simulink model "pfb_legacy"  (Simulink 6.2)
settings: Solver=ode45  StartTime=0.0  StopTime=40000  RelTol=1e-3
undefined symbols (not defined in the file): BEE2_usr
libraries: xbsIndex_r3 x189, xps_library x42, adcscope_lib x6, pfb_library x3, fft_library x3, correlator_library x3
(part 2 of 2)

== system pfb_legacy/data_mux_in/tvg ==
  note: BRAM READ/WRITE MUX
      | lspitler - 13 Jan 09
      | Simplified TVG
      | tvg_ctrl sets 'length', 'skip', 'stall'
  Constant : xbsIndex_r3/Constant  const=0  equ=P=C  arith_type=Unsigned  n_bits=32  bin_pt=0  opselect=C  inp2=PCIN>>17  opr=+  inp1=P  carry=CIN  iostate=0  explicit_period=on  period=1  dbl_ovrd=off
  Constant1 : xbsIndex_r3/Constant  const=0  equ=P=C  arith_type=Unsigned  n_bits=32  bin_pt=0  opselect=C  inp2=PCIN>>17  opr=+  inp1=P  carry=CIN  iostate=0  explicit_period=on  period=1  dbl_ovrd=off
  Constant2 : xbsIndex_r3/Constant  const=0  equ=P=C  arith_type=Boolean  n_bits=32  bin_pt=0  opselect=C  inp2=PCIN>>17  opr=+  inp1=P  carry=CIN  iostate=0  explicit_period=on  period=1  dbl_ovrd=off
  Constant3 : xbsIndex_r3/Constant  const=0  equ=P=C  arith_type=Boolean  n_bits=32  bin_pt=0  opselect=C  inp2=PCIN>>17  opr=+  inp1=P  carry=CIN  iostate=0  explicit_period=on  period=1  dbl_ovrd=off
  ram_im : xps_library/Shared BRAM  Tag=xps:bram  arith_type="Signed  (2's comp)"  addr_width=11  data_width=32  data_bin_pt=0  init_vals=[1:2^11]  sample_rate=1
  ram_re : xps_library/Shared BRAM  Tag=xps:bram  arith_type="Signed  (2's comp)"  addr_width=11  data_width=32  data_bin_pt=0  init_vals=[1:2^11]  sample_rate=1
  thr_cpu_ctrl_sim : Subsystem  mask{tvg_skip=1, tvg_stall=1, tvg_length=512}
      mask prompts: tvg_skip "Skip"; tvg_stall "Stall"; tvg_length "Length"
      mask help:
      | Mux Data for CT and FFT Syncs:
      |
      | 0 -> Interchip Connection
      | 1 -> User Generated External Sync
      | 2 -> Periodic Sync Generator
      | 3 -> Periodic Sync Generator (Same as 2)
      |
      | Mux Data for CT and FFT Inputs:
      |
      | 0 -> Interchip Connection
      | 1 -> Test Vector Generator (TVG)
      | 2 -> All Zeroes (0's)
      | 3 -> All Ones (1's)
  tvg : Subsystem  mask(Test Vector Generator(TVG)){tvg_skip=1, tvg_stall=1, tvg_length=512}
      mask prompts: tvg_skip "Skip"; tvg_stall "Stall"; tvg_length "Length"
  tvg_ctrl : xps_library/software register  Tag=xps:sw_reg  io_dir=From Processor  arith_type=Unsigned  bitwidth=32  bin_pt=0  sample_period=1  gw_name=pfb_legacy_data_mux_in_tvg_tvg_ctrl_user_data_out
  re_out : Outport
  im_out : Outport  Port=2
  wires:
  ram_im/1 -> im_out/1
  ram_re/1 -> re_out/1
  thr_cpu_ctrl_sim/1(out) -> tvg_ctrl/1
  tvg_ctrl/1 -> tvg/1(In1)
  tvg/1(Out1) -> ram_im/1, ram_re/1
  Constant/1 -> ram_re/2
  Constant1/1 -> ram_im/2
  Constant2/1 -> ram_re/3
  Constant3/1 -> ram_im/3

== system pfb_legacy/data_out_mux/tvg ==
  note: BRAM READ/WRITE MUX
      | lspitler - 13 Jan 09
      | Simplified TVG
      | tvg_ctrl sets 'length', 'skip', 'stall'
  Constant : xbsIndex_r3/Constant  const=0  equ=P=C  arith_type=Unsigned  n_bits=32  bin_pt=0  opselect=C  inp2=PCIN>>17  opr=+  inp1=P  carry=CIN  iostate=0  explicit_period=on  period=1  dbl_ovrd=off
  Constant1 : xbsIndex_r3/Constant  const=0  equ=P=C  arith_type=Unsigned  n_bits=32  bin_pt=0  opselect=C  inp2=PCIN>>17  opr=+  inp1=P  carry=CIN  iostate=0  explicit_period=on  period=1  dbl_ovrd=off
  Constant2 : xbsIndex_r3/Constant  const=0  equ=P=C  arith_type=Boolean  n_bits=32  bin_pt=0  opselect=C  inp2=PCIN>>17  opr=+  inp1=P  carry=CIN  iostate=0  explicit_period=on  period=1  dbl_ovrd=off
  Constant3 : xbsIndex_r3/Constant  const=0  equ=P=C  arith_type=Boolean  n_bits=32  bin_pt=0  opselect=C  inp2=PCIN>>17  opr=+  inp1=P  carry=CIN  iostate=0  explicit_period=on  period=1  dbl_ovrd=off
  ram_im : xps_library/Shared BRAM  Tag=xps:bram  arith_type="Signed  (2's comp)"  addr_width=11  data_width=32  data_bin_pt=0  init_vals=[1:2^11]  sample_rate=1
  ram_re : xps_library/Shared BRAM  Tag=xps:bram  arith_type="Signed  (2's comp)"  addr_width=11  data_width=32  data_bin_pt=0  init_vals=[1:2^11]  sample_rate=1
  thr_cpu_ctrl_sim : Subsystem  mask{tvg_skip=1, tvg_stall=2, tvg_length=5}
      mask prompts: tvg_skip "Skip"; tvg_stall "Stall"; tvg_length "Length"
      mask help:
      | Mux Data for CT and FFT Syncs:
      |
      | 0 -> Interchip Connection
      | 1 -> User Generated External Sync
      | 2 -> Periodic Sync Generator
      | 3 -> Periodic Sync Generator (Same as 2)
      |
      | Mux Data for CT and FFT Inputs:
      |
      | 0 -> Interchip Connection
      | 1 -> Test Vector Generator (TVG)
      | 2 -> All Zeroes (0's)
      | 3 -> All Ones (1's)
  tvg : Subsystem  mask(Test Vector Generator(TVG)){tvg_skip=1, tvg_stall=1, tvg_length=512}
      mask prompts: tvg_skip "Skip"; tvg_stall "Stall"; tvg_length "Length"
  tvg_ctrl : xps_library/software register  Tag=xps:sw_reg  io_dir=From Processor  arith_type=Unsigned  bitwidth=32  bin_pt=0  sample_period=1  gw_name=pfb_legacy_data_out_mux_tvg_tvg_ctrl_user_data_out
  re_out : Outport
  im_out : Outport  Port=2
  wires:
  ram_im/1 -> im_out/1
  ram_re/1 -> re_out/1
  thr_cpu_ctrl_sim/1(out) -> tvg_ctrl/1
  tvg_ctrl/1 -> tvg/1(In1)
  tvg/1(Out1) -> ram_im/1, ram_re/1
  Constant/1 -> ram_re/2
  Constant1/1 -> ram_im/2
  Constant2/1 -> ram_re/3
  Constant3/1 -> ram_im/3

== system pfb_legacy/data_mux_in/tvg/thr_cpu_ctrl_sim ==
  Concat : xbsIndex_r3/Concat  num_inputs=4  explicit_period=off  period=1  dbl_ovrd=off
  Delay : xbsIndex_r3/Delay  latency=1  reg_retiming=off  explicit_period=off  period=1  en=off  accept_only_valid=off  init_zero=on  dbl_ovrd=off  show_param=off
      settings: xl_area=[0, 0, 0, 0, 0, 0, 0]
  Disregard Subsystem : xbsIndex_r3/Disregard Subsystem  Tag=discardX
      settings: AttributesFormatString=Disregard Subsystem\nFor Generation
  Gateway Out : xbsIndex_r3/Gateway Out  output_type=Double  nbits=8  bin_pt=6  arith_type=Boolean  quantization=Truncate  overflow=Wrap  hdl_port=off  timing_constraint=None  locs_specified=off  LOCs={}  needs_fixed_name=off  show_param=off
      settings: xl_area=[0, 0, 0, 0, 0, 0, 0]
  Length : xbsIndex_r3/Constant  const=tvg_length  equ=P=C  arith_type=Unsigned  n_bits=10  bin_pt=0  opselect=C  inp2=PCIN>>17  opr=+  inp1=P  carry=CIN  iostate=0  explicit_period=on  period=1  dbl_ovrd=off
  "Skip\t" : xbsIndex_r3/Constant  const=tvg_skip  equ=P=C  arith_type=Unsigned  n_bits=10  bin_pt=0  opselect=C  inp2=PCIN>>17  opr=+  inp1=P  carry=CIN  iostate=0  explicit_period=on  period=1  dbl_ovrd=off
  Stall : xbsIndex_r3/Constant  const=tvg_stall  equ=P=C  arith_type=Unsigned  n_bits=10  bin_pt=0  opselect=C  inp2=PCIN>>17  opr=+  inp1=P  carry=CIN  iostate=0  explicit_period=on  period=1  dbl_ovrd=off
  pad_zeroes : xbsIndex_r3/Constant  const=0  equ=P=C  arith_type=Unsigned  n_bits=2  bin_pt=0  opselect=C  inp2=PCIN>>17  opr=+  inp1=P  carry=CIN  iostate=0  explicit_period=on  period=1  dbl_ovrd=off
  out : Outport
  wires:
  Length/1 -> Concat/2
  pad_zeroes/1 -> Concat/1
  Stall/1 -> Concat/3
  Gateway Out/1 -> out/1
  Concat/1 -> Delay/1
  Delay/1 -> Gateway Out/1
  "Skip\t"/1 -> Concat/4

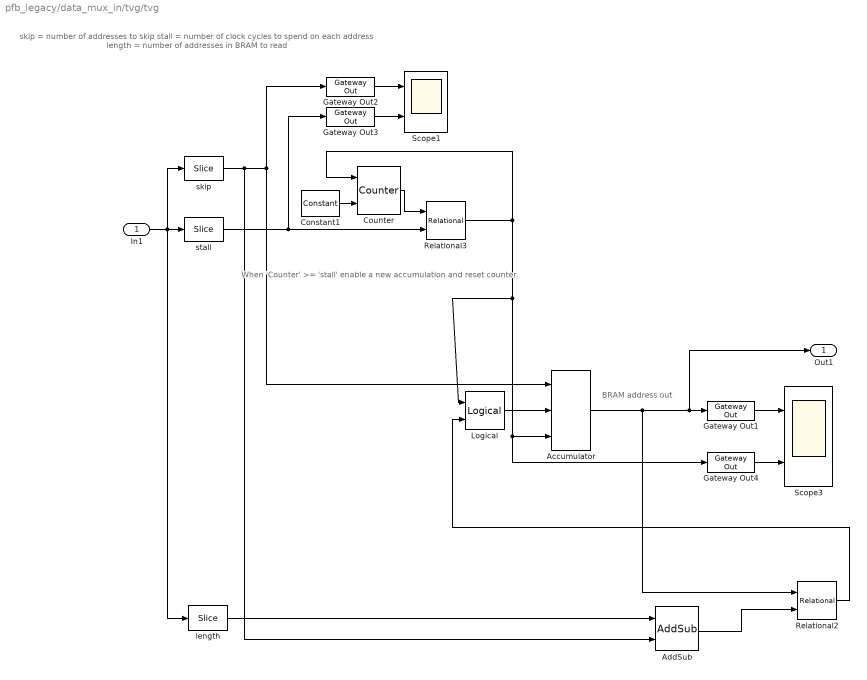
== system pfb_legacy/data_mux_in/tvg/tvg ==
  note: BRAM address out
  note: When 'Counter' >= 'stall'
      | enable a new accumulation
      | and reset counter.
  note: skip = number of addresses to skip
      | stall = number of clock cycles to spend
      | on each address
      | length = number of addresses in BRAM
      | to read
  In1 : Inport  Port=1  LatchInput=off
  Accumulator : xbsIndex_r3/Accumulator  n_bits=10  overflow=Wrap  operation=Add  scale=1  explicit_period=on  period=1  rst=on  hasbypass=off  en=on  dbl_ovrd=off  show_param=off  gen_core=off  use_rpm=on
      settings: xl_area=[0, 0, 0, 0, 0, 0, 0]
  AddSub : xbsIndex_r3/AddSub  mode=Subtraction  precision=Full  arith_type=Unsigned  n_bits=8  bin_pt=2  quantization=Truncate  overflow=Wrap  latency=1  explicit_period=on  period=1  use_carryin=off  use_carryout=off  en=off  dbl_ovrd=off  show_param=off  use_core=on  pipeline=off  use_rpm=on  gen_core=off
      settings: xl_area=[0, 0, 0, 0, 0, 0, 0]
  Constant1 : xbsIndex_r3/Constant  const=1  equ=P=C  arith_type=Unsigned  n_bits=10  bin_pt=0  opselect=C  inp2=PCIN>>17  opr=+  inp1=P  carry=CIN  iostate=0  explicit_period=on  period=1  dbl_ovrd=off
  Counter : xbsIndex_r3/Counter  cnt_type=Free Running  n_bits=10  bin_pt=0  arith_type=Unsigned  start_count=0  cnt_to=inf  cnt_by_val=1  operation=Up  explicit_period=on  period=1  load_pin=on  rst=off  en=off  dbl_ovrd=off  show_param=off  use_rpm=on  gen_core=off
      settings: xl_area=[0, 0, 0, 0, 0, 0, 0]
  Gateway Out{1..4} (4 alike) : xbsIndex_r3/Gateway Out  output_type=Double  nbits=8  bin_pt=6  arith_type=Boolean  quantization=Truncate  overflow=Wrap  hdl_port=on  timing_constraint=None  locs_specified=off  LOCs={}  needs_fixed_name=off  show_param=off
      settings: xl_area=[0, 0, 0, 0, 0, 0, 0]
  Logical : xbsIndex_r3/Logical  logical_function=AND  inputs=2  precision=Full  arith_type=Unsigned  n_bits=8  bin_pt=2  align_bp=on  latency=0  explicit_period=off  period=1  en=off  dbl_ovrd=off  show_param=off
      settings: xl_area=[0, 0, 0, 0, 0, 0, 0]
  Relational2 : xbsIndex_r3/Relational  mode=a>=b  latency=0  explicit_period=on  period=1  en=off  dbl_ovrd=off  show_param=off
      settings: xl_area=[0, 0, 0, 0, 0, 0, 0]
  Relational3 : xbsIndex_r3/Relational  mode=a>=b  latency=0  explicit_period=on  period=1  en=off  dbl_ovrd=off  show_param=off
      settings: xl_area=[0, 0, 0, 0, 0, 0, 0]
  Scope1 : Scope  NumInputPorts=2
      settings: YMin=-5~-5  YMax=5~5
  Scope3 : Scope  NumInputPorts=2
      settings: TimeRange=20  YMin=-5~-5  YMax=5~5  SaveName=ScopeData4
  length : xbsIndex_r3/Slice  mode=Lower Bit Location + Width  nbits=10  bit1=0  base1=MSB of Input  bit0=20  base0=LSB of Input  boolean_output=off  explicit_period=on  period=1  dbl_ovrd=off
  skip : xbsIndex_r3/Slice  mode=Lower Bit Location + Width  nbits=10  bit1=0  base1=MSB of Input  bit0=0  base0=LSB of Input  boolean_output=off  explicit_period=on  period=1  dbl_ovrd=off
  stall : xbsIndex_r3/Slice  mode=Lower Bit Location + Width  nbits=10  bit1=0  base1=MSB of Input  bit0=10  base0=LSB of Input  boolean_output=off  explicit_period=on  period=1  dbl_ovrd=off
  Out1 : Outport
  wires:
  In1/1 -> stall/1, skip/1, length/1
  Gateway Out1/1 -> Scope3/1
  Accumulator/1 -> Gateway Out1/1, Out1/1, Relational2/1
  skip/1 -> Gateway Out2/1, Accumulator/1, AddSub/2
  stall/1 -> Gateway Out3/1, Relational3/2
  Gateway Out2/1 -> Scope1/1
  Gateway Out3/1 -> Scope1/2
  Gateway Out4/1 -> Scope3/2
  Relational3/1 -> Counter/1, Accumulator/3, Gateway Out4/1, Logical/1
  Counter/1 -> Relational3/1
  Constant1/1 -> Counter/2
  Relational2/1 -> Logical/2
  Logical/1 -> Accumulator/2
  length/1 -> AddSub/1
  AddSub/1 -> Relational2/2

== system pfb_legacy/data_out_mux/tvg/thr_cpu_ctrl_sim ==
  Concat : xbsIndex_r3/Concat  num_inputs=4  explicit_period=off  period=1  dbl_ovrd=off
  Delay : xbsIndex_r3/Delay  latency=1  reg_retiming=off  explicit_period=off  period=1  en=off  accept_only_valid=off  init_zero=on  dbl_ovrd=off  show_param=off
      settings: xl_area=[0, 0, 0, 0, 0, 0, 0]
  Disregard Subsystem : xbsIndex_r3/Disregard Subsystem  Tag=discardX
      settings: AttributesFormatString=Disregard Subsystem\nFor Generation
  Gateway Out : xbsIndex_r3/Gateway Out  output_type=Double  nbits=8  bin_pt=6  arith_type=Boolean  quantization=Truncate  overflow=Wrap  hdl_port=off  timing_constraint=None  locs_specified=off  LOCs={}  needs_fixed_name=off  show_param=off
      settings: xl_area=[0, 0, 0, 0, 0, 0, 0]
  Length : xbsIndex_r3/Constant  const=tvg_length  equ=P=C  arith_type=Unsigned  n_bits=10  bin_pt=0  opselect=C  inp2=PCIN>>17  opr=+  inp1=P  carry=CIN  iostate=0  explicit_period=on  period=1  dbl_ovrd=off
  "Skip\t" : xbsIndex_r3/Constant  const=tvg_skip  equ=P=C  arith_type=Unsigned  n_bits=10  bin_pt=0  opselect=C  inp2=PCIN>>17  opr=+  inp1=P  carry=CIN  iostate=0  explicit_period=on  period=1  dbl_ovrd=off
  Stall : xbsIndex_r3/Constant  const=tvg_stall  equ=P=C  arith_type=Unsigned  n_bits=10  bin_pt=0  opselect=C  inp2=PCIN>>17  opr=+  inp1=P  carry=CIN  iostate=0  explicit_period=on  period=1  dbl_ovrd=off
  pad_zeroes : xbsIndex_r3/Constant  const=0  equ=P=C  arith_type=Unsigned  n_bits=2  bin_pt=0  opselect=C  inp2=PCIN>>17  opr=+  inp1=P  carry=CIN  iostate=0  explicit_period=on  period=1  dbl_ovrd=off
  out : Outport
  wires:
  Length/1 -> Concat/2
  pad_zeroes/1 -> Concat/1
  Stall/1 -> Concat/3
  Gateway Out/1 -> out/1
  Concat/1 -> Delay/1
  Delay/1 -> Gateway Out/1
  "Skip\t"/1 -> Concat/4

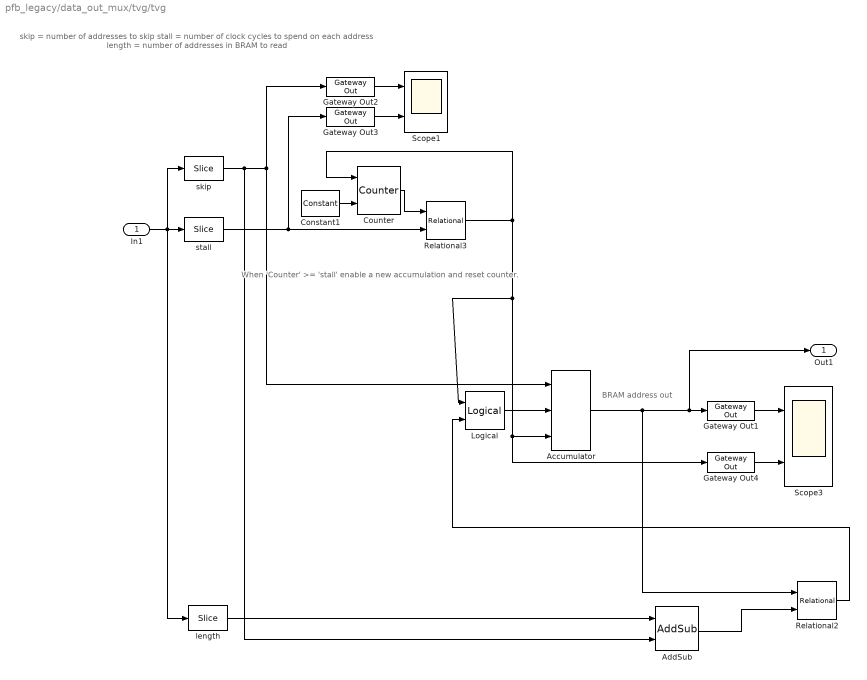
== system pfb_legacy/data_out_mux/tvg/tvg ==
  note: BRAM address out
  note: When 'Counter' >= 'stall'
      | enable a new accumulation
      | and reset counter.
  note: skip = number of addresses to skip
      | stall = number of clock cycles to spend
      | on each address
      | length = number of addresses in BRAM
      | to read
  In1 : Inport  Port=1  LatchInput=off
  Accumulator : xbsIndex_r3/Accumulator  n_bits=10  overflow=Wrap  operation=Add  scale=1  explicit_period=on  period=1  rst=on  hasbypass=off  en=on  dbl_ovrd=off  show_param=off  gen_core=off  use_rpm=on
      settings: xl_area=[0, 0, 0, 0, 0, 0, 0]
  AddSub : xbsIndex_r3/AddSub  mode=Subtraction  precision=Full  arith_type=Unsigned  n_bits=8  bin_pt=2  quantization=Truncate  overflow=Wrap  latency=1  explicit_period=on  period=1  use_carryin=off  use_carryout=off  en=off  dbl_ovrd=off  show_param=off  use_core=on  pipeline=off  use_rpm=on  gen_core=off
      settings: xl_area=[0, 0, 0, 0, 0, 0, 0]
  Constant1 : xbsIndex_r3/Constant  const=1  equ=P=C  arith_type=Unsigned  n_bits=10  bin_pt=0  opselect=C  inp2=PCIN>>17  opr=+  inp1=P  carry=CIN  iostate=0  explicit_period=on  period=1  dbl_ovrd=off
  Counter : xbsIndex_r3/Counter  cnt_type=Free Running  n_bits=10  bin_pt=0  arith_type=Unsigned  start_count=0  cnt_to=inf  cnt_by_val=1  operation=Up  explicit_period=on  period=1  load_pin=on  rst=off  en=off  dbl_ovrd=off  show_param=off  use_rpm=on  gen_core=off
      settings: xl_area=[0, 0, 0, 0, 0, 0, 0]
  Gateway Out{1..4} (4 alike) : xbsIndex_r3/Gateway Out  output_type=Double  nbits=8  bin_pt=6  arith_type=Boolean  quantization=Truncate  overflow=Wrap  hdl_port=on  timing_constraint=None  locs_specified=off  LOCs={}  needs_fixed_name=off  show_param=off
      settings: xl_area=[0, 0, 0, 0, 0, 0, 0]
  Logical : xbsIndex_r3/Logical  logical_function=AND  inputs=2  precision=Full  arith_type=Unsigned  n_bits=8  bin_pt=2  align_bp=on  latency=0  explicit_period=off  period=1  en=off  dbl_ovrd=off  show_param=off
      settings: xl_area=[0, 0, 0, 0, 0, 0, 0]
  Relational2 : xbsIndex_r3/Relational  mode=a>=b  latency=0  explicit_period=on  period=1  en=off  dbl_ovrd=off  show_param=off
      settings: xl_area=[0, 0, 0, 0, 0, 0, 0]
  Relational3 : xbsIndex_r3/Relational  mode=a>=b  latency=0  explicit_period=on  period=1  en=off  dbl_ovrd=off  show_param=off
      settings: xl_area=[0, 0, 0, 0, 0, 0, 0]
  Scope1 : Scope  NumInputPorts=2
      settings: YMin=-5~-5  YMax=5~5
  Scope3 : Scope  NumInputPorts=2
      settings: TimeRange=20  YMin=-5~-5  YMax=5~5  SaveName=ScopeData4
  length : xbsIndex_r3/Slice  mode=Lower Bit Location + Width  nbits=10  bit1=0  base1=MSB of Input  bit0=20  base0=LSB of Input  boolean_output=off  explicit_period=on  period=1  dbl_ovrd=off
  skip : xbsIndex_r3/Slice  mode=Lower Bit Location + Width  nbits=10  bit1=0  base1=MSB of Input  bit0=0  base0=LSB of Input  boolean_output=off  explicit_period=on  period=1  dbl_ovrd=off
  stall : xbsIndex_r3/Slice  mode=Lower Bit Location + Width  nbits=10  bit1=0  base1=MSB of Input  bit0=10  base0=LSB of Input  boolean_output=off  explicit_period=on  period=1  dbl_ovrd=off
  Out1 : Outport
  wires:
  In1/1 -> stall/1, skip/1, length/1
  Gateway Out1/1 -> Scope3/1
  Accumulator/1 -> Gateway Out1/1, Out1/1, Relational2/1
  skip/1 -> Gateway Out2/1, Accumulator/1, AddSub/2
  stall/1 -> Gateway Out3/1, Relational3/2
  Gateway Out2/1 -> Scope1/1
  Gateway Out3/1 -> Scope1/2
  Gateway Out4/1 -> Scope3/2
  Relational3/1 -> Counter/1, Accumulator/3, Gateway Out4/1, Logical/1
  Counter/1 -> Relational3/1
  Constant1/1 -> Counter/2
  Relational2/1 -> Logical/2
  Logical/1 -> Accumulator/2
  length/1 -> AddSub/1
  AddSub/1 -> Relational2/2
